simulink model "EENG447"  (R2025b)
settings: Solver=ode23tb  StartTime=0.0  StopTime=25  MaxStep=5e-05  RelTol=1e-3
libraries: spsSeriesRLCBranchLib x3, spsUniversalBridgeLib x2, spsAsynchronousMachinepuUnitsLib x1, spsIGBTLib x1, spsPWMGenerator2LevelLib x1, simulink x1, spsThreePhaseSourceLib x1, spsVoltageMeasurementLib x1, sps_lib x1
settings Model: SimulationMode=rapid-accelerator  Creator=sayedali  LastModifiedBy=sayedali

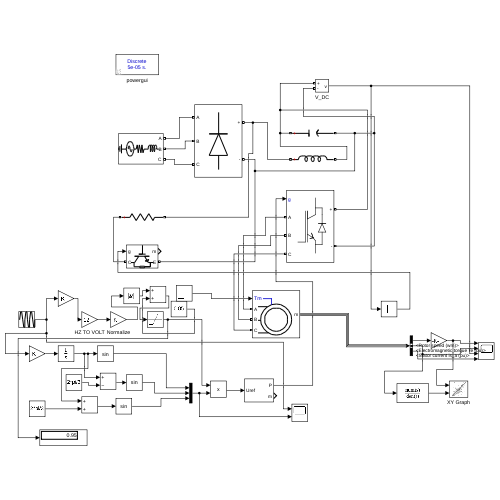
[thumbnail: Simulink's stored preview of the top-level diagram]
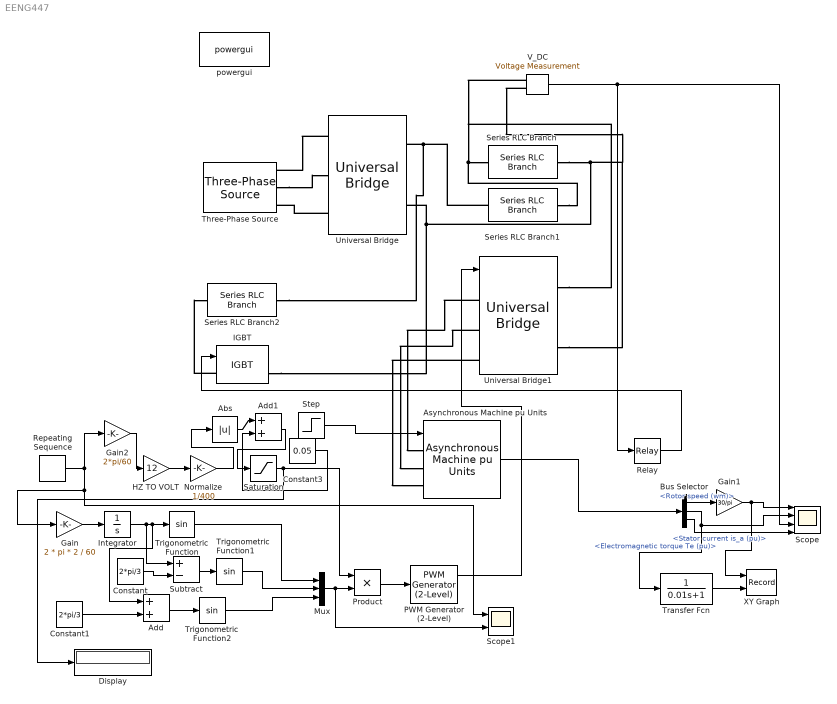
== system EENG447 ==
  Abs : Abs  SaturateOnIntegerOverflow=off
  Add : Sum
  Add1 : Sum
  Asynchronous Machine pu Units : spsAsynchronousMachinepuUnitsLib/Asynchronous Machine pu Units  RotorType=Squirrel-cage  PresetModel="15:  5.4 HP (4KW)   400 V  50Hz 1430 RPM"  MechanicalLoad=Torque Tm  ShowDetailedParameters=on  ReferenceFrame=Rotor  Units=pu  MeasurementBus=off  NominalParameters=[4000 400 50]  VoltageRatio=1  Stator=[0.03513 0.04586]  Rotor=[0.03488 0.04586]  Cage1=[0.01909 0.0397]  Cage2=[0.01909 0.0397]  Lm=1.352  Mechanical=[0.0404 0.01841 2]  PolePairs=2  InitialConditions="[ 1,0   0,0,0   0,0,0 ]"  SimulateSaturation=off  Saturation="[0.212,0.4201,0.8125,1.0979,1.4799,2.2457,3.2586,4.5763,6.4763 ;   0.5,0.7,0.9,1,1.1,1.2 ,1.3,1.4,1.5]"  LoadFlowParameters=0  TsPowergui=0  TsBlock=-1  IterativeModel=Trapezoidal non iterative  IterativeDiscreteModel=Trapezoidal non iterative  Pmec=0
      settings: LibrarySourceBlock=|
      | sps_lib/Electrical Machines/Asynchronous Machine
      | pu Units
  Bus Selector : BusSelector  OutputSignals=Mechanical.Rotor speed (wm),Mechanical.Electromagnetic torque Te (pu),Stator measurements.Stator current is_a (pu)
  Constant : Constant  Value=2*pi/3
  Constant1 : Constant  Value=2*pi/3
  Constant3 : Constant  Value=0.05
  Display : Display
  Gain : Gain  Gain=2 * pi * 2 / 60
  Gain1 : Gain  Gain=30/pi
  Gain2 : Gain  Gain=2*pi/60
  HZ TO VOLT : Gain  Gain=12
  IGBT : spsIGBTLib/IGBT  Ron=0.001  Lon=0  Vf=1  Tf=1e-6  Tt=2e-6  IC=0  Rs=1e5  Cs=inf  Measurements=on
  Integrator : Integrator
  Mux : Mux  Inputs=3
  Normalize : Gain  Gain=1/400
  PWM Generator (2-Level) : spsPWMGenerator2LevelLib/PWM Generator (2-Level)  ModulatorType=Three-phase bridge (6 pulses)  ModulatorMode=Unsynchronized  Fc=1000  Pc=90  nF=27  MinMax="[ -1  1 ]"  SamplingTechnique=Natural  ModulatingSignals=off  m=0.8  Freq=60  Phase=0  Ts=5e-05  ShowCarrierOutport=on
  Product : Product
  Relay : Relay  OnSwitchValue=700  OffSwitchValue=650
  Repeating Sequence : simulink/Sources/Repeating Sequence  rep_seq_t=[0 4 8 12 16 20]  rep_seq_y=[0 1500 1500 0 -1500 -1500]
  Saturation : Saturate  UpperLimit=0.95  LowerLimit=0
  Scope : Scope  NumInputPorts=4
      settings: ActiveDisplayYMinimum=-13.698628460576153  ActiveDisplayYMaximum=12.179909859934224
  Scope1 : Scope  NumInputPorts=2
      settings: ActiveDisplayYMinimum=-1875  ActiveDisplayYMaximum=1875
  Series RLC Branch : spsSeriesRLCBranchLib/Series RLC Branch  LConnTagsString=__new0  RConnTagsString=__new0  BranchType=C  Resistance=1  Inductance=1e-3  SetiL0=off  InitialCurrent=0  Capacitance=2200e-6  Setx0=off  InitialVoltage=0  Measurements=None
  Series RLC Branch1 : spsSeriesRLCBranchLib/Series RLC Branch  LConnTagsString=__new0  RConnTagsString=__new0  BranchType=L  Resistance=1  Inductance=1e-3  SetiL0=off  InitialCurrent=0  Capacitance=1e-6  Setx0=off  InitialVoltage=0  Measurements=None
  Series RLC Branch2 : spsSeriesRLCBranchLib/Series RLC Branch  LConnTagsString=__new0  RConnTagsString=__new0  BranchType=R  Resistance=60  Inductance=1e-3  SetiL0=off  InitialCurrent=0  Capacitance=1e-6  Setx0=off  InitialVoltage=0  Measurements=None
  Step : Step  After=0.75  SampleTime=0
  Subtract : Sum  Inputs=+-
  Three-Phase Source : spsThreePhaseSourceLib/Three-Phase Source  InternalConnection=Yg  VoltagePhases=off  Voltage=500  PhaseAngle=0  Voltage_phases=[25e3 25e3 25e3]/sqrt(3)  PhaseAngles_phases=[0 -120 +120]  Frequency=50  NonIdealSource=on  SpecifyImpedance=off  Resistance=0.8929  Inductance=16.58e-3  ShortCircuitLevel=100e6  BaseVoltage=25e3  XRratio=7  BusType=swing  Pref=10e3  Qref=0  Prefabc=[10e3, 10e3, 10e3]  Qrefabc=[0, 0, 0]  Qmin=-inf  Qmax=inf
  Transfer Fcn : TransferFcn  Denominator=[0.01 1]
  Trigonometric Function : Trigonometry
  Trigonometric Function1 : Trigonometry
  Trigonometric Function2 : Trigonometry
  Universal Bridge : spsUniversalBridgeLib/Universal Bridge  Arms=3  SnubberResistance=1e5  SnubberCapacitance=inf  Device=Diodes  Ron=1e-3  Lon=0  ForwardVoltages="[  0  0  ]"  ForwardVoltage=0  GTOparameters=[ 10e-6 , 20e-6 ]  IGBTparameters=[ 1e-6 , 2e-6 ]  Measurements=None  Measurements_2=None  converterType=Rectifier
  Universal Bridge1 : spsUniversalBridgeLib/Universal Bridge  Arms=3  SnubberResistance=1e5  SnubberCapacitance=inf  Device=IGBT / Diodes  Ron=1e-3  Lon=0  ForwardVoltages="[  0  0  ]"  ForwardVoltage=0  GTOparameters=[ 10e-6 , 20e-6 ]  IGBTparameters=[ 1e-6 , 2e-6 ]  Measurements=None  Measurements_2=None  converterType=Rectifier
  V_DC : spsVoltageMeasurementLib/Voltage Measurement  PhasorSimulation=off  OutputType=Complex  PSBequivalent=0
  XY Graph : Record  NumPorts=2.0  FileSettingsInternal="{\"entries\":[{\"content\":{\"excelSettings\":{\"content\":{},\"type\":\"Streamout.ExcelSettings\"},\"parquetSettings\":{\"content\":{},\"type\":\"Streamout.ParquetSettings\"}},\"type\":\"Streamout.FileSettingStorage\",\"uuid\":\"\"}],\"packageUris\":[\"http:\\/\\/schema.mathworks.com\\/mf0\\/streamout_blocks\\/R2020a\"],\"version\":\"1.0\"}"  FrameSettings=[0, 0]  Layout=[1 1]  SignalsInternal="{\"entries\":[{\"content\":{\"signals\":[{\"content\":{\"blockPath\":[],\"dimensions\":[1],\"domain\":\"\",\"lineColor\":\"#a2142f\",\"plots\":[ 1 ],\"port\":1,\"sid\":[\"\"],\"signalID\":1,\"signalName\":\"Gain1\"},\"type\":\"RecordBlkView.Signal\",\"uuid\":\"\"},{\"content\":{\"blockPath\":[],\"dimensions\":[1],\"domain\":\"\",\"lineColor\":\"#139fff\",\"plots\":[ 1 ],\"port\":2,\"sid\":[\"\"],\"signalID\":2,\"signalName\":\"Transfer Fcn\"},\"type\":\"RecordBlkView.Signal\",\"uuid\":\"\"}]},\"type\":\"RecordBlkView.InputSignals\",\"uuid\":\"\"}],\"packageUris\":[\"http:\\/\\/schema.mathworks.com\\/mf0\\/streamout_blocks\\/R2020a\"],\"version\":\"1.0\"}"  VisualizationBindings="{\"xyplotplugin\":{\"info\":[{\"series\":[{\"bindingParametersList\":[{\"parameter\":\"X-Axis\",\"signalID\":1,\"signalName\":\"Gain1\"},{\"parameter\":\"Y-Axis\",\"signalID\":2,\"signalName\":\"Transfer Fcn\"}],\"seriesID\":0}],\"subplotID\":1}]}}"  CompatibilityTag=XY
  powergui : sps_lib/powergui  Priority=1  SimulationMode=Discrete  SampleTime=5e-05  frequency=60  Iterations=50  frequencyindice=50  Pbase=100e6  ErrMax=1e-4  UnitsV=kV  UnitsW=MW  buscounter=0  FunctionMessages=off  echomessages=off  EnableUseOfTLC=off  CurrentSourceSwitches=off  DisableSnubberDevices=off  DisableRonSwitches=off  DisableVfSwitches=off  DisplayEquations=off  AutomaticDiscreteSolvers=off  SolverType=Tustin/Backward Euler (TBE)  Interpol=off  ExternalGateDelay=off  methode=off  Ts=100  x0status=blocks  SPID=on  SwTol=0  HookPort=off  NonlinearTolerance=1e-4  nMaxIteration=100  ContinueOnMaxIteration=off  RestoreLinks=warning  ResistiveCurrentMeasurement=off  Frange=[0:2:500]  Ylog=off  Xlog=on  ShowGrid=off  save=off  variable=ZData  structure=0  ZoomFFT=off  StartTime=0.0  cycles=1  DisplayStyle=1  fundamental=60  FreqAxis=off  MaxFrequency=1000  frequencyindicesteady=1  RmsSteady=1  display=off
  wires:
  HZ TO VOLT/1 -> Normalize/1
  Gain/1 -> Integrator/1
  Integrator/1 -> Subtract/1, Add/1, Trigonometric Function/1
  Constant/1 -> Subtract/2
  Subtract/1 -> Trigonometric Function1/1
  Constant1/1 -> Add/2
  Add/1 -> Trigonometric Function2/1
  Trigonometric Function/1 -> Mux/1
  Trigonometric Function1/1 -> Mux/2
  Trigonometric Function2/1 -> Mux/3
  Mux/1 -> Scope1/2, Product/2
  Saturation/1 -> Display/1, Product/1
  Product/1 -> PWM Generator (2-Level)/1
  PWM Generator (2-Level)/1 -> Universal Bridge1/1
  Relay/1 -> IGBT/1
  V_DC/1 -> Scope/3, Relay/1
  Asynchronous Machine pu Units/1 -> Bus Selector/1
  Bus Selector/1 -> Gain1/1  "<Rotor speed (wm)>"
  Gain1/1 -> XY Graph/1, Scope/1
  Bus Selector/2 -> Transfer Fcn/1, Scope/2  "<Electromagnetic torque Te (pu)>"
  Gain2/1 -> HZ TO VOLT/1
  Bus Selector/3 -> Scope/4  "<Stator current is_a (pu)>"
  Step/1 -> Asynchronous Machine pu Units/1
  Normalize/1 -> Abs/1
  Repeating Sequence/1 -> Scope1/1, Gain/1, Gain2/1
  Abs/1 -> Add1/1
  Constant3/1 -> Add1/2
  Add1/1 -> Saturation/1
  Transfer Fcn/1 -> XY Graph/2
  connections:
  Universal Bridge/LConn1 -- Three-Phase Source/RConn1
  Three-Phase Source/RConn2 -- Universal Bridge/LConn2
  Universal Bridge/LConn3 -- Three-Phase Source/RConn3
  Series RLC Branch1/LConn1 -- Series RLC Branch2/RConn1 -- Universal Bridge/RConn1
  Series RLC Branch1/RConn1 -- V_DC/LConn1 -- Universal Bridge1/RConn1 -- Series RLC Branch/LConn1
  Series RLC Branch/RConn1 -- V_DC/LConn2 -- Universal Bridge1/RConn2 -- IGBT/RConn1 -- Universal Bridge/RConn2
  IGBT/LConn1 -- Series RLC Branch2/LConn1
  Universal Bridge1/LConn3 -- Asynchronous Machine pu Units/LConn3
  Universal Bridge1/LConn1 -- Asynchronous Machine pu Units/LConn1
  Universal Bridge1/LConn2 -- Asynchronous Machine pu Units/LConn2
